simulink model "ballbeam_sim"  (Simulink 8.3)
settings: Solver=ode45  StartTime=0.0  StopTime=1000  RelTol=1e-3
undefined symbols (not defined in the file or in its folder): AP, drawBallBeam
settings Model: Creator=beard  LastModifiedBy=jhl48
settings OptimizationCC: ExpressionDepthLimit=2147483647  InitFltsAndDblsToZero=on
settings DebuggingCC: FcnCallInpInsideContextMsg=UseLocalSettings

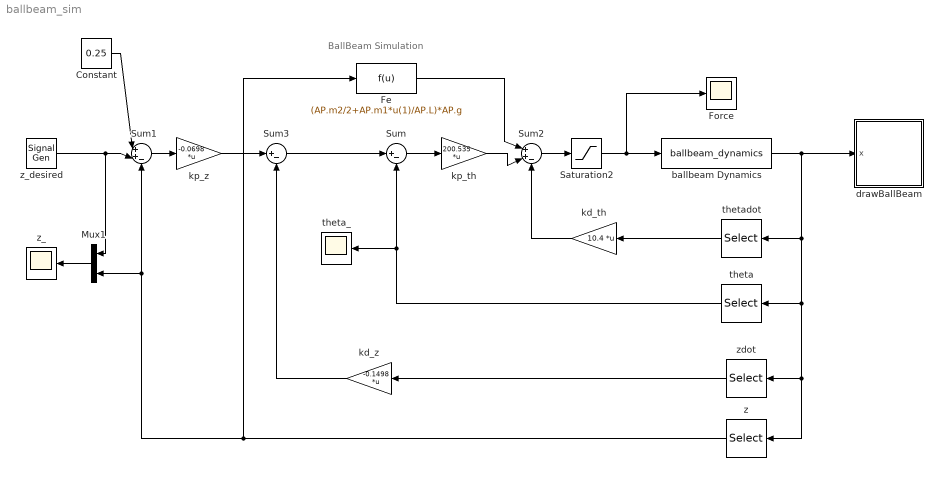
== system ballbeam_sim ==
  note: BallBeam Simulation
  Constant : Constant  Value=0.25
  Fe : Fcn  Expr=(AP.m2/2+AP.m1*u(1)/AP.L)*AP.g
  Force : Scope
      settings: TimeRange=100  YMin=7  YMax=15
  Mux1 : Mux  Inputs=2
  Saturation2 : Saturate  UpperLimit=15  LowerLimit=-15
  Sum : Sum  Inputs=|+-
  Sum1 : Sum  Inputs=|++-
  Sum2 : Sum  Inputs=|++-
  Sum3 : Sum  Inputs=|+-
  ballbeam Dynamics : S-Function  FunctionName=ballbeam_dynamics  Parameters=AP  EnableBusSupport=off
  drawBallBeam : Subsystem
      mask init:
      | % drawing parameters
      | L = .5;
      | R = L/10;
      mask Display: image(imread('tv.jpg'))
  kd_th : Gain  Gain=10.4  Multiplication=Matrix(K*u)
  kd_z : Gain  Gain=-0.1498  Multiplication=Matrix(K*u)
  kp_th : Gain  Gain=200.535  Multiplication=Matrix(K*u)
  kp_z : Gain  Gain=-0.0698  Multiplication=Matrix(K*u)
  theta : Selector  InputPortWidth=4  Indices=[1]
  theta_ : Scope
      settings: TimeRange=100  YMin=-0.02  YMax=0.0225
  thetadot : Selector  InputPortWidth=4  Indices=[3]
  z : Selector  InputPortWidth=4  Indices=[2]
  z_ : Scope
      settings: TimeRange=100  YMin=-0.15  YMax=0.4  SaveName=ScopeData2
  z_desired : SignalGenerator  WaveForm=square  Amplitude=0.125  Frequency=.1
  zdot : Selector  InputPortWidth=4  Indices=[4]
  wires:
  ballbeam Dynamics/1 -> drawBallBeam/1(x), theta/1, z/1, zdot/1, thetadot/1
  Sum2/1 -> Saturation2/1
  Sum/1 -> kp_th/1
  theta/1 -> Sum/2, theta_/1
  z/1 -> Fe/1, Sum1/3, Mux1/2
  z_desired/1 -> Mux1/1, Sum1/2
  Mux1/1 -> z_/1
  thetadot/1 -> kd_th/1
  Sum1/1 -> kp_z/1
  kp_z/1 -> Sum3/1
  zdot/1 -> kd_z/1
  kd_z/1 -> Sum3/2
  Sum3/1 -> Sum/1
  kd_th/1 -> Sum2/3
  kp_th/1 -> Sum2/2
  Saturation2/1 -> ballbeam Dynamics/1, Force/1
  Fe/1 -> Sum2/1
  Constant/1 -> Sum1/1

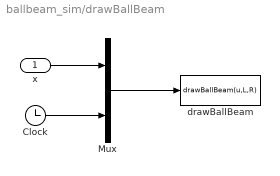
== system ballbeam_sim/drawBallBeam ==
  x : Inport
  Clock : Clock
  Mux : Mux  Inputs=2
  drawBallBeam : MATLABFcn  MATLABFcn=drawBallBeam(u,L,R)  OutputDimensions=0  SampleTime=0.01
  wires:
  Mux/1 -> drawBallBeam/1
  x/1 -> Mux/1
  Clock/1 -> Mux/2
